simulink model "FCS"  (Simulink 9.1)
settings: Solver=VariableStepAuto  StartTime=0.0  StopTime=10.0  RelTol=1e-3
values from neighbouring files (symbols this model uses):
  Controller =     [data_set.mat]
  Estimator =     [data_set.mat]
  g = 9.81    [data_set.mat]
  init =     [data_set.mat]
  Sensors =     [data_set.mat]
  Ts = 0.005    [data_set.mat]
  Vehicle =     [data_set.mat]
undefined symbols (not defined in the file or in its folder): DiscIntNeverNeededParam, Discrete, Time
libraries: F_Line_block x470, simulink x33, ctrlSharedLib x3, sharedtransform x3, sharedutil x1
(part 3 of 3)

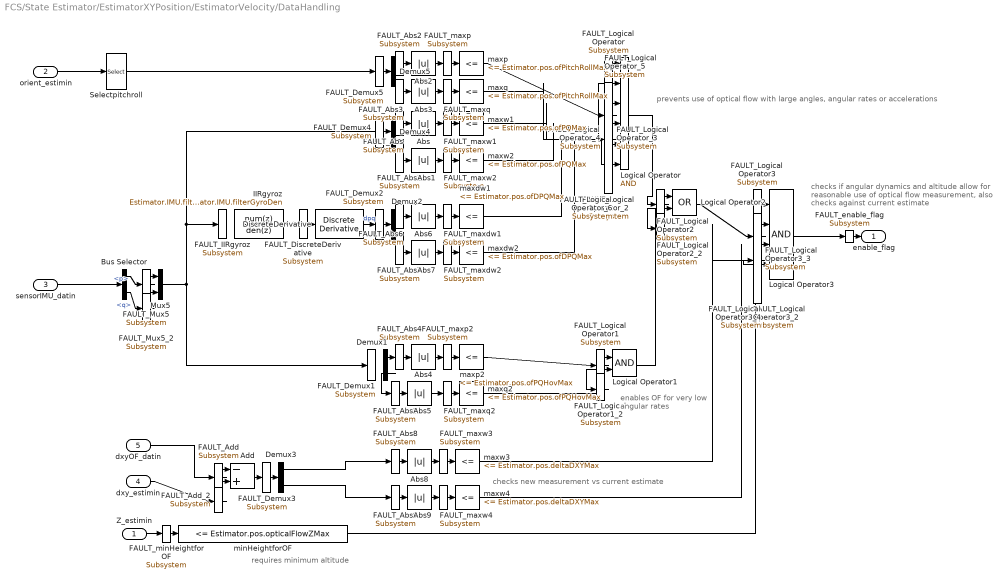
== system FCS/State Estimator/EstimatorXYPosition/EstimatorVelocity/DataHandling ==
  note: prevents use of optical flow with large angles, angular rates or accelerations
  note: enables OF for very
      | low angular rates
  note: checks if angular dynamics and altitude allow for
      | reasonable use of optical flow measurement,
      | also checks against current estimate
  note: checks new measurement vs current estimate
  note: requires minimum altitude
  Z_estimin : Inport
  orient_estimin : Inport  Port=2
  sensorIMU_datin : Inport  Port=3
  dxy_estimin : Inport  Port=4
  dxyOF_datin : Inport  Port=5
  Abs{,1..9} (10 alike) : Abs
  FAULT_Abs{,1..9} (10 alike) : F_Line_block/Subsystem
  Add : Sum  Inputs=-+
  FAULT_Add : F_Line_block/Subsystem
  FAULT_Add_2 : F_Line_block/Subsystem
  Bus Selector : BusSelector  OutputSignals=p,q
  Demux{1..5} (5 alike) : Demux  Outputs=2
  FAULT_Demux{1..5} (5 alike) : F_Line_block/Subsystem
  DiscreteDerivative : simulink/Discrete/Discrete Derivative  gainval=1.0  ICPrevScaledInput=0.0  InputProcessing=Inherited  OutMin=[]  OutMax=[]  OutDataType=fixdt(1, 16)  OutScaling=2^-10  DoSatur=off
  FAULT_DiscreteDerivative : F_Line_block/Subsystem
  IIRgyroz : DiscreteFilter  Numerator=Estimator.IMU.filterGyroNum  Denominator=Estimator.IMU.filterGyroDen
  FAULT_IIRgyroz : F_Line_block/Subsystem
  Logical Operator : Logic  Inputs=6  AllPortsSameDT=off  OutDataTypeStr=boolean
  FAULT_Logical Operator{,1..3} (4 alike) : F_Line_block/Subsystem
  FAULT_Logical Operator_{2..6} (5 alike) : F_Line_block/Subsystem
  Logical Operator1 : Logic  AllPortsSameDT=off  OutDataTypeStr=boolean
  FAULT_Logical Operator1_2 : F_Line_block/Subsystem
  Logical Operator2 : Logic  Operator=OR  AllPortsSameDT=off  OutDataTypeStr=boolean
  FAULT_Logical Operator2_2 : F_Line_block/Subsystem
  Logical Operator3 : Logic  Inputs=4  AllPortsSameDT=off  OutDataTypeStr=boolean
  FAULT_Logical Operator3_2 : F_Line_block/Subsystem
  FAULT_Logical Operator3_3 : F_Line_block/Subsystem
  FAULT_Logical Operator3_4 : F_Line_block/Subsystem
  Mux5 : Mux  Inputs=2
  FAULT_Mux5 : F_Line_block/Subsystem
  FAULT_Mux5_2 : F_Line_block/Subsystem
  Selectpitchroll : Selector  InputPortWidth=3  IndexOptions=Index vector (dialog)  Indices=[2 3]  OutputSizes=1
  maxdw1 : simulink/Logic and Bit Operations/Compare To Constant  relop=<=  const=Estimator.pos.ofDPQMax  OutDataTypeStr=boolean
  FAULT_maxdw1 : F_Line_block/Subsystem
  maxdw2 : simulink/Logic and Bit Operations/Compare To Constant  relop=<=  const=Estimator.pos.ofDPQMax  OutDataTypeStr=boolean
  FAULT_maxdw2 : F_Line_block/Subsystem
  maxp : simulink/Logic and Bit Operations/Compare To Constant  relop=<=  const=Estimator.pos.ofPitchRollMax  OutDataTypeStr=boolean
  FAULT_maxp : F_Line_block/Subsystem
  maxp2 : simulink/Logic and Bit Operations/Compare To Constant  relop=<=  const=Estimator.pos.ofPQHovMax  OutDataTypeStr=boolean
  FAULT_maxp2 : F_Line_block/Subsystem
  maxq : simulink/Logic and Bit Operations/Compare To Constant  relop=<=  const=Estimator.pos.ofPitchRollMax  OutDataTypeStr=boolean
  FAULT_maxq : F_Line_block/Subsystem
  maxq2 : simulink/Logic and Bit Operations/Compare To Constant  relop=<=  const=Estimator.pos.ofPQHovMax  OutDataTypeStr=boolean
  FAULT_maxq2 : F_Line_block/Subsystem
  maxw1 : simulink/Logic and Bit Operations/Compare To Constant  relop=<=  const=Estimator.pos.ofPQMax  OutDataTypeStr=boolean
  FAULT_maxw{1..4} (4 alike) : F_Line_block/Subsystem
  maxw2 : simulink/Logic and Bit Operations/Compare To Constant  relop=<=  const=Estimator.pos.ofPQMax  OutDataTypeStr=boolean
  maxw3 : simulink/Logic and Bit Operations/Compare To Constant  relop=<=  const=Estimator.pos.deltaDXYMax  OutDataTypeStr=boolean
  maxw4 : simulink/Logic and Bit Operations/Compare To Constant  relop=<=  const=Estimator.pos.deltaDXYMax  OutDataTypeStr=boolean
  minHeightforOF : simulink/Logic and Bit Operations/Compare To Constant  relop=<=  const=Estimator.pos.opticalFlowZMax  OutDataTypeStr=boolean
  FAULT_minHeightforOF : F_Line_block/Subsystem
  enable_flag : Outport
  FAULT_enable_flag : F_Line_block/Subsystem
  wires:
  minHeightforOF/1 -> FAULT_Logical Operator3_4/1
  FAULT_Logical Operator3_4/1 -> Logical Operator3/4
  IIRgyroz/1 -> FAULT_DiscreteDerivative/1
  FAULT_DiscreteDerivative/1 -> DiscreteDerivative/1
  Mux5/1 -> FAULT_Demux1/1, FAULT_IIRgyroz/1, Demux4/1
  maxw4/1 -> FAULT_Logical Operator3_3/1
  FAULT_Logical Operator3_3/1 -> Logical Operator3/3
  maxw3/1 -> FAULT_Logical Operator3_2/1
  FAULT_Logical Operator3_2/1 -> Logical Operator3/2
  dxyOF_datin/1 -> FAULT_Add/1
  FAULT_Add/1 -> Add/1
  Demux3/2 -> FAULT_Abs9/1
  FAULT_Abs9/1 -> Abs9/1
  Demux3/1 -> FAULT_Abs8/1
  FAULT_Abs8/1 -> Abs8/1
  dxy_estimin/1 -> FAULT_Add_2/1
  FAULT_Add_2/1 -> Add/2
  Add/1 -> FAULT_Demux3/1
  FAULT_Demux3/1 -> Demux3/1
  Abs9/1 -> FAULT_maxw4/1
  FAULT_maxw4/1 -> maxw4/1
  Abs8/1 -> FAULT_maxw3/1
  FAULT_maxw3/1 -> maxw3/1
  Logical Operator2/1 -> FAULT_Logical Operator3/1
  FAULT_Logical Operator3/1 -> Logical Operator3/1
  Logical Operator3/1 -> FAULT_enable_flag/1
  FAULT_enable_flag/1 -> enable_flag/1
  DiscreteDerivative/1 -> FAULT_Demux2/1  "dpq"
  FAULT_Demux2/1 -> Demux2/1
  Demux2/2 -> FAULT_Abs7/1
  FAULT_Abs7/1 -> Abs7/1
  Demux2/1 -> FAULT_Abs6/1
  FAULT_Abs6/1 -> Abs6/1
  Abs7/1 -> FAULT_maxdw2/1
  FAULT_maxdw2/1 -> maxdw2/1
  Abs6/1 -> FAULT_maxdw1/1
  FAULT_maxdw1/1 -> maxdw1/1
  Logical Operator1/1 -> FAULT_Logical Operator2_2/1
  FAULT_Logical Operator2_2/1 -> Logical Operator2/2
  Demux1/2 -> FAULT_Abs5/1
  FAULT_Abs5/1 -> Abs5/1
  Demux1/1 -> FAULT_Abs4/1
  FAULT_Abs4/1 -> Abs4/1
  Abs5/1 -> FAULT_maxq2/1
  FAULT_maxq2/1 -> maxq2/1
  Abs4/1 -> FAULT_maxp2/1
  FAULT_maxp2/1 -> maxp2/1
  Abs3/1 -> FAULT_maxq/1
  FAULT_maxq/1 -> maxq/1
  Abs2/1 -> FAULT_maxp/1
  FAULT_maxp/1 -> maxp/1
  Demux4/2 -> FAULT_Abs1/1
  FAULT_Abs1/1 -> Abs1/1
  Demux4/1 -> FAULT_Abs/1
  FAULT_Abs/1 -> Abs/1
  Abs1/1 -> FAULT_maxw2/1
  FAULT_maxw2/1 -> maxw2/1
  Abs/1 -> FAULT_maxw1/1
  FAULT_maxw1/1 -> maxw1/1
  Z_estimin/1 -> FAULT_minHeightforOF/1
  FAULT_minHeightforOF/1 -> minHeightforOF/1
  Logical Operator/1 -> FAULT_Logical Operator2/1
  FAULT_Logical Operator2/1 -> Logical Operator2/1
  maxw1/1 -> FAULT_Logical Operator_3/1
  FAULT_Logical Operator_3/1 -> Logical Operator/3
  Bus Selector/1 -> FAULT_Mux5/1  "<p>"
  FAULT_Mux5/1 -> Mux5/1
  Selectpitchroll/1 -> FAULT_Demux5/1
  FAULT_Demux5/1 -> Demux5/1
  sensorIMU_datin/1 -> Bus Selector/1
  maxq2/1 -> FAULT_Logical Operator1_2/1
  FAULT_Logical Operator1_2/1 -> Logical Operator1/2
  Bus Selector/2 -> FAULT_Mux5_2/1  "<q>"
  FAULT_Mux5_2/1 -> Mux5/2
  maxp/1 -> FAULT_Logical Operator/1
  FAULT_Logical Operator/1 -> Logical Operator/1
  maxw2/1 -> FAULT_Logical Operator_4/1
  FAULT_Logical Operator_4/1 -> Logical Operator/4
  orient_estimin/1 -> Selectpitchroll/1
  maxdw1/1 -> FAULT_Logical Operator_5/1
  FAULT_Logical Operator_5/1 -> Logical Operator/5
  maxdw2/1 -> FAULT_Logical Operator_6/1
  FAULT_Logical Operator_6/1 -> Logical Operator/6
  maxq/1 -> FAULT_Logical Operator_2/1
  FAULT_Logical Operator_2/1 -> Logical Operator/2
  Demux5/1 -> FAULT_Abs2/1
  FAULT_Abs2/1 -> Abs2/1
  Demux5/2 -> FAULT_Abs3/1
  FAULT_Abs3/1 -> Abs3/1
  maxp2/1 -> FAULT_Logical Operator1/1
  FAULT_Logical Operator1/1 -> Logical Operator1/1

== system FCS/State Estimator/EstimatorXYPosition/EstimatorXYPosition/OutlierHandling ==
  orient_estimin : Inport
  posVIS_datin : Inport  Port=2
  pos_estim : Inport  Port=3
  Abs : Abs
  FAULT_Abs : F_Line_block/Subsystem
  Abs1 : Abs
  FAULT_Abs1 : F_Line_block/Subsystem
  Add1 : Sum  Inputs=+-  AccumDataTypeStr=single
  FAULT_Add1 : F_Line_block/Subsystem
  FAULT_Add1_2 : F_Line_block/Subsystem
  Constant : Constant  Value=2  OutDataTypeStr=single
  Demux : Demux  Outputs=2
  FAULT_Demux : F_Line_block/Subsystem
  Logical Operator3 : Logic  Inputs=4  AllPortsSameDT=off  OutDataTypeStr=boolean
  FAULT_Logical Operator3 : F_Line_block/Subsystem
  FAULT_Logical Operator3_2 : F_Line_block/Subsystem
  FAULT_Logical Operator3_3 : F_Line_block/Subsystem
  FAULT_Logical Operator3_4 : F_Line_block/Subsystem
  Math Function : Math  Operator=pow  SaturateOnIntegerOverflow=on
  FAULT_Math Function : F_Line_block/Subsystem
  FAULT_Math Function_2 : F_Line_block/Subsystem
  SelectX : Selector  InputPortWidth=4  IndexOptions=Index vector (dialog)  Indices=[1]  OutputSizes=1
  SelectXY : Selector  InputPortWidth=4  IndexOptions=Index vector (dialog)  Indices=[1 2]  OutputSizes=1
  Selector : Selector  InputPortWidth=3  IndexOptions=Index vector (dialog)  Indices=[2 3]  OutputSizes=1
  Sqrt : Sqrt  SaturateOnIntegerOverflow=on
  FAULT_Sqrt : F_Line_block/Subsystem
  Sum of Elements : Sum  Inputs=+
  FAULT_Sum of Elements : F_Line_block/Subsystem
  checkifPosavailable : simulink/Logic and Bit Operations/Compare To Constant  relop=~=  const=-99  OutDataTypeStr=boolean
  FAULT_checkifPosavailable : F_Line_block/Subsystem
  maxp3 : simulink/Logic and Bit Operations/Compare To Constant  relop=<=  const=Estimator.pos.visOrientMax  OutDataTypeStr=boolean
  FAULT_maxp3 : F_Line_block/Subsystem
  maxq3 : simulink/Logic and Bit Operations/Compare To Constant  relop=<=  const=Estimator.pos.visOrientMax  OutDataTypeStr=boolean
  FAULT_maxq3 : F_Line_block/Subsystem
  planarjumpsVISPOS : simulink/Logic and Bit Operations/Compare To Constant  relop=<  const=Estimator.pos.visDeltaXYMax  OutDataTypeStr=boolean
  FAULT_planarjumpsVISPOS : F_Line_block/Subsystem
  enable_flag : Outport
  FAULT_enable_flag : F_Line_block/Subsystem
  wires:
  Abs1/1 -> FAULT_maxq3/1
  FAULT_maxq3/1 -> maxq3/1
  Abs/1 -> FAULT_maxp3/1
  FAULT_maxp3/1 -> maxp3/1
  Demux/2 -> FAULT_Abs1/1
  FAULT_Abs1/1 -> Abs1/1
  Demux/1 -> FAULT_Abs/1
  FAULT_Abs/1 -> Abs/1
  Selector/1 -> FAULT_Demux/1
  FAULT_Demux/1 -> Demux/1
  orient_estimin/1 -> Selector/1
  planarjumpsVISPOS/1 -> FAULT_Logical Operator3_4/1
  FAULT_Logical Operator3_4/1 -> Logical Operator3/4
  Sqrt/1 -> FAULT_planarjumpsVISPOS/1
  FAULT_planarjumpsVISPOS/1 -> planarjumpsVISPOS/1
  pos_estim/1 -> FAULT_Add1_2/1
  FAULT_Add1_2/1 -> Add1/2
  Add1/1 -> FAULT_Math Function/1
  FAULT_Math Function/1 -> Math Function/1
  SelectXY/1 -> FAULT_Add1/1
  FAULT_Add1/1 -> Add1/1
  maxq3/1 -> FAULT_Logical Operator3_3/1
  FAULT_Logical Operator3_3/1 -> Logical Operator3/3
  maxp3/1 -> FAULT_Logical Operator3_2/1
  FAULT_Logical Operator3_2/1 -> Logical Operator3/2
  Logical Operator3/1 -> FAULT_enable_flag/1
  FAULT_enable_flag/1 -> enable_flag/1
  checkifPosavailable/1 -> FAULT_Logical Operator3/1
  FAULT_Logical Operator3/1 -> Logical Operator3/1
  SelectX/1 -> FAULT_checkifPosavailable/1
  FAULT_checkifPosavailable/1 -> checkifPosavailable/1
  posVIS_datin/1 -> SelectX/1, SelectXY/1
  Sum of Elements/1 -> FAULT_Sqrt/1
  ?FAULT_Demux1/1 -> ?Demux1/1
  ?FAULT_IIRgyroz/1 -> ?IIRgyroz/1
  FAULT_Sqrt/1 -> Sqrt/1
  Constant/1 -> FAULT_Math Function_2/1
  FAULT_Math Function_2/1 -> Math Function/2
  Math Function/1 -> FAULT_Sum of Elements/1
  FAULT_Sum of Elements/1 -> Sum of Elements/1
